simulink model "P3_model"  (R2018b)
settings: Solver=VariableStepAuto  StartTime=0.0  StopTime=2  RelTol=1e-3
values from neighbouring files (symbols this model uses):
  A = (2 - 3.7887*T) * (2 + 3.9791*T) / 2 / (2 + 10.2083*T)    (= 0.429666937991)    [P3.m]    (also in Transfer.m = [0, 1, 0; 15.0757, -0.1904, 13.1260; 0, 0, -250])
  C1 = (-2-3.7887*T) / (2-3.7887*T)    (= -2.2199378552)    [P3.m]
  C2 = (-2 + 3.9791*T) / (2 + 3.9791*T)    (= -0.430707270139)    [P3.m]
  C3 = (-2 + 10.2083*T) / (2 + 10.2083*T)    (= 0.0103076458683)    [P3.m]
  K_M = 19.0620 * (-1 - p(1)) * (-1 - p(2)) / (-1 - z(1)) / (-1 - z(2))    [P3.m]
  T = 0.2    [P3.m]
settings Model: Creator=hadiz  LastModifiedBy=hadiz

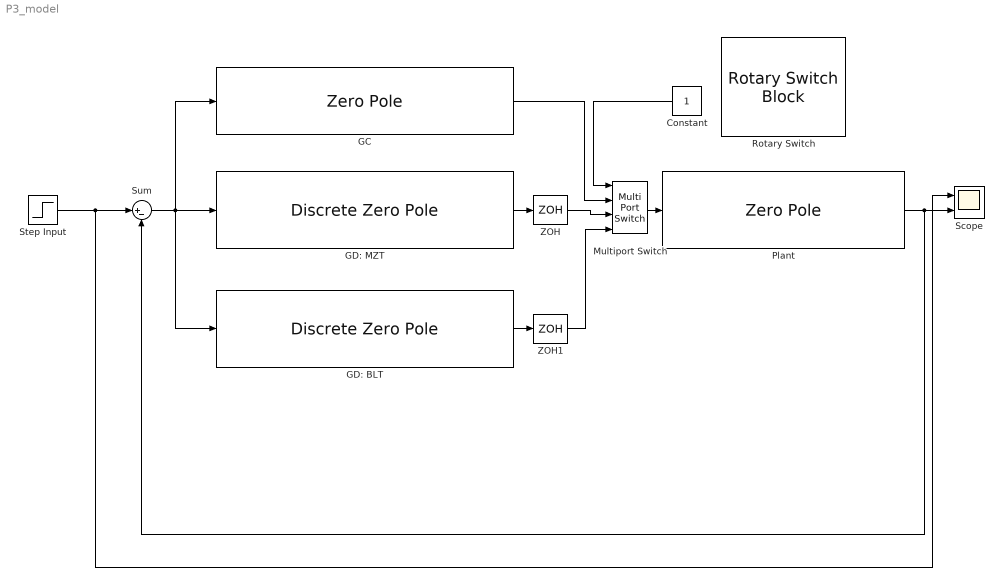
== system P3_model ==
  Constant : Constant
  GC : ZeroPole  Zeros=[3.7887, -3.9791]  Poles=[0, -10.2083]  Gain=19.0620
  GD: BLT : DiscreteZeroPole  Zeros=[-C1, -C2]  Poles=[1, -C3]  Gain=19.0620 * A  SampleTime=T
  GD: MZT : DiscreteZeroPole  Zeros=[exp(3.7887*T), exp(-3.9791*T)]  Poles=[1, exp(-10.2083*T)]  Gain=K_M  SampleTime=T
  Multiport Switch : MultiPortSwitch
  Plant : ZeroPole  Zeros=[]  Poles=[-250, -3.9791, +3.7887]  Gain=656.3
  Rotary Switch : RotarySwitchBlock  WebBlockId=25
      settings: Values={{'GC', 'GD: MZT', 'GD: BLT'}, [1 2 3]}
  Scope : Scope  NumInputPorts=2
  "Step Input " : Step  Time=0  SampleTime=0
  Sum : Sum  Inputs=|+-
  ZOH : ZeroOrderHold  SampleTime=T
  ZOH1 : ZeroOrderHold  SampleTime=T
  wires:
  GD: MZT/1 -> ZOH/1
  Sum/1 -> GD: BLT/1, GC/1, GD: MZT/1
  Plant/1 -> Sum/2, Scope/2
  "Step Input "/1 -> Scope/1, Sum/1
  GD: BLT/1 -> ZOH1/1
  Multiport Switch/1 -> Plant/1
  ZOH1/1 -> Multiport Switch/4
  ZOH/1 -> Multiport Switch/3
  GC/1 -> Multiport Switch/2
  Constant/1 -> Multiport Switch/1
